simulink model "Qube"  (R2020b)
settings: Solver=VariableStepAuto  StartTime=0.0  StopTime=10  MaxStep=1.0  RelTol=1e-3
InitFcn:
  | if libisloaded('pid')
  |     unloadlibrary('pid')
  | end
  | loadlibrary('../C/src/pid.so','../C/src/PID.h')
  | 
  | if calllib('pid','initialize','dataPID.bin') ~= 0
  |       error('couble not load PID');
  | end
  | 
  | 
  | load('Qube','G'); % Load model
libraries: cstblocks x1
CloseFcn:
  | unloadlibrary('pid')
settings Model: Creator=philippe  LastModifiedBy=philippe
settings HardwareCC: TargetBitPerPointer=64  TargetBitPerSizeT=64  TargetBitPerPtrDiffT=64  TargetLargestAtomicFloat=Float  TargetIntDivRoundTo=Zero  TargetEndianess=LittleEndian  TargetWordSize=64  TargetHWDeviceType=Intel->x86-64 (Windows64)
settings SFSimCC: SimParseCustomCode=off

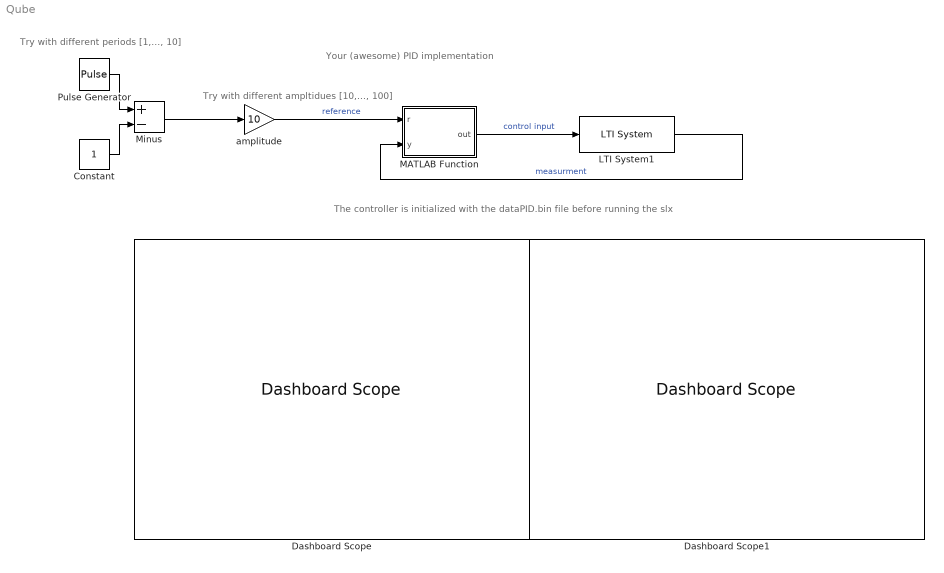
== system Qube ==
  note: The controller is initialized with the dataPID.bin file before running the slx
  note: Your (awesome) PID implementation
  note: Try with different ampltidues [10,..., 100]
  note: Try with different periods [1,..., 10]
  Constant : Constant
  Dashboard Scope : DashboardScope
  Dashboard Scope1 : DashboardScope
  LTI System1 : cstblocks/LTI System  sys=G  IC=[]
  MATLAB Function : MATLAB Function  TreatAsAtomicUnit=on
  Minus : Sum  Inputs=+-
  Pulse Generator : DiscretePulseGenerator  PulseType=Time based  Amplitude=2  Period=4  PulseWidth=50
  amplitude : Gain  Gain=10
  wires:
  LTI System1/1 -> MATLAB Function/2(y)  "measurment"
  MATLAB Function/1(out) -> LTI System1/1  "control input"
  amplitude/1 -> MATLAB Function/1(r)  "reference"
  Pulse Generator/1 -> Minus/1
  Minus/1 -> amplitude/1
  Constant/1 -> Minus/2

== matlab function Qube/MATLAB Function ==
  data: r input; y input; out output
function out = calcPID(r,y)
% wrapper around the calc function
coder.extrinsic('calcPID');
 
out = 0; % tell MATLAB out is a double
out = calcPID(y,r);

end
